simulink model "poly3DoublyNormalized"  (R2023b)
settings: Solver=FixedStepAuto  StartTime=0.0  StopTime=10  FixedStep=0.0001  MaxStep=0.001  RelTol=1e-3
settings Model: Creator=ggi01  LastModifiedBy=ggi01
settings SolverCC: AlgebraicLoopSolver=TrustRegion
settings DebuggingCC: UnconnectedInputMsg=warning  UnconnectedOutputMsg=warning  UnconnectedLineMsg=warning
settings ModelReferenceCC: EnableRefExpFcnMdlSchedulingChecks=on
settings RTWCC: DLArmComputeVersion=19.05

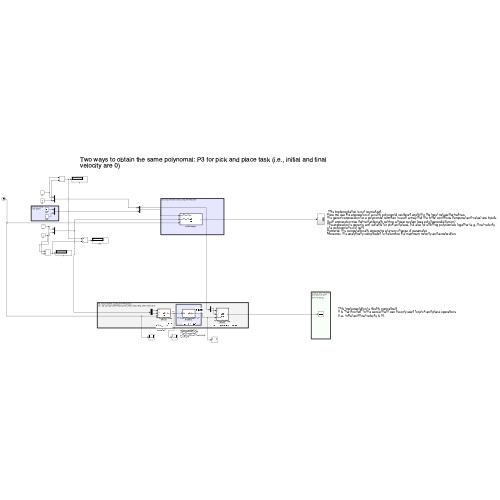
[thumbnail: Simulink's stored preview of the top-level diagram]
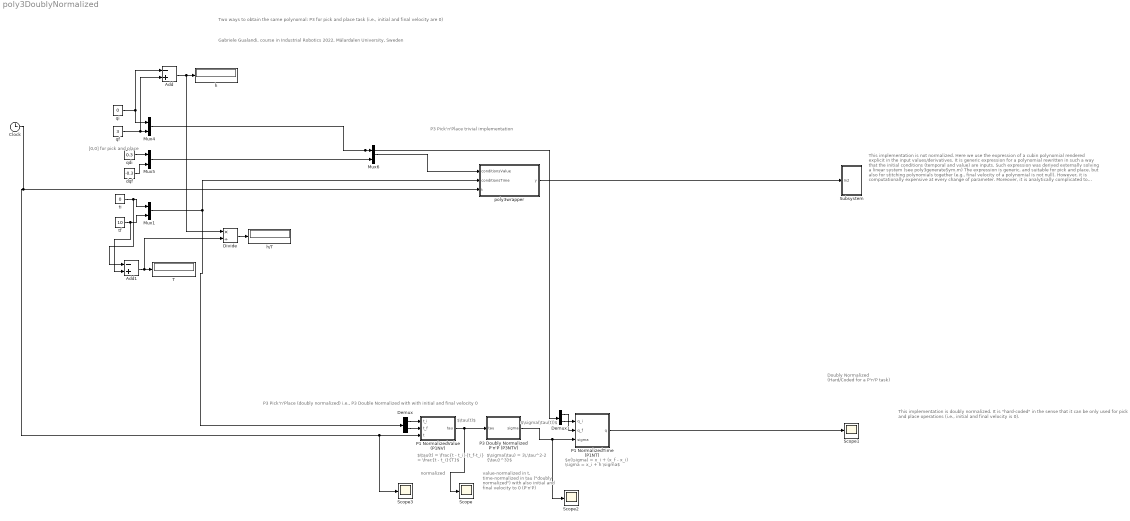
== system poly3DoublyNormalized ==
  note: P3 Pick'n'Place trivial implementation
  note: Gabriele Gualandi, course in Industrial Robotics 2022, Mälardalen University, Sweden
  note: normalized
  note: Two ways to obtain the same polynomal: P3 for pick and place task (i.e., initial and final velocity are 0)
  note: [0,0] for pick
      | and place
  note: P3 Pick'n'Place (doubly normalized)
      | i.e., P3 Double Normalized with with initial and final velocity 0
  note: Doubly Normalized
      | (Hard/Coded for
      | a P'n'P task)
  note: This implementation is not normalized.
      | Here we use the expression of a cubin polynomial rendered explicit in the input values/derivatives.
      | It is generic expression for a polynomial rewritten in such a way that the initial conditions (temporal and value) are inputs. Such expression was derived externally solving a linear system (see poly3generateSym.m)
      | The expression is generic, and suitable for pick and place, but also for stitching polynomials together (e.g., final velocity of a polynomial is not null).
      | However, it is computationally expensive at every change of parameter.
      | Moreover, it is analytically complicated to determine the maximum velocity and acceleration.
  note: This implementation is doubly normalized.
      | It is "hard-coded" in the sense that it can be only used for pick and place operations
      | (i.e., initial and final velocity is 0).
  note: $\sigma(\tau) = 3\,\tau^2-2 {\tau}^3}$
  note: $\tau(t)$
  note: value-normalized in t,
      | time-normalized in tau
      | ("doubly normalized")
      | with also initial and final velocity
      | to 0 (P'n'P)
  note: $\sigma(\tau(t))$
  note: $\tau(t) = \frac{t - t_i}{t_f-t_i} = \frac{t - t_i}{T}$
  note: $x(\sigma) = x_i + (x_f - x_i) \sigma = x_i + h \sigma$
  Add : Sum  Inputs=-+
  Add1 : Sum  Inputs=-+
  Clock : Clock
  Demux : Demux  Outputs=2
  Demux1 : Demux  Outputs=2
  Divide : Product  Inputs=*/
  Mux{1,4..6} (4 alike) : Mux  Inputs=2
  P1 NormalizedTime (P1NT) : MATLAB Function  TreatAsAtomicUnit=on
  P1 NormalizedValue (P1NV) : MATLAB Function  TreatAsAtomicUnit=on
  P3 Doubly Normalized P'n'P (P3NTV) : MATLAB Function  TreatAsAtomicUnit=on
  Scope{,1..3} (4 alike) : Scope
  Subsystem : Subsystem
  T : Display
  dqf : Constant  Value=-0.3
  h : Display
  h/T : Display
  poly3wrapper : MATLAB Function  TreatAsAtomicUnit=on
  qdi : Constant  Value=0.3
  qf : Constant  Value=3
  qi : Constant  Value=0
  tf : Constant  Value=10
  ti : Constant  Value=0
  wires:
  qi/1 -> Mux4/1, Add/1
  qf/1 -> Add/2, Mux4/2
  qdi/1 -> Mux5/1
  dqf/1 -> Mux5/2
  ti/1 -> Add1/1, Mux1/1
  tf/1 -> Add1/2, Mux1/2
  Mux1/1 -> Demux/1, poly3wrapper/2(conditionsTime)
  Mux4/1 -> Demux1/1, Mux6/1
  Mux6/1 -> poly3wrapper/1(conditionsValue)
  Mux5/1 -> Mux6/2
  Demux/1 -> P1 NormalizedValue (P1NV)/1(t_i)
  Demux/2 -> P1 NormalizedValue (P1NV)/2(t_f)
  Demux1/1 -> P1 NormalizedTime (P1NT)/1(q_i)
  Demux1/2 -> P1 NormalizedTime (P1NT)/2(q_f)
  P1 NormalizedTime (P1NT)/1(q) -> Scope1/1
  P1 NormalizedValue (P1NV)/1(tau) -> Scope/1, P3 Doubly Normalized P'n'P (P3NTV)/1(tau)
  P3 Doubly Normalized P'n'P (P3NTV)/1(sigma) -> Scope2/1, P1 NormalizedTime (P1NT)/3(sigma)
  Clock/1 -> Scope3/1, P1 NormalizedValue (P1NV)/3(t), poly3wrapper/3(t)
  poly3wrapper/1(y) -> Subsystem/1(In2)
  Add/1 -> Divide/1, h/1
  Add1/1 -> Divide/2, T/1
  Divide/1 -> h/T/1

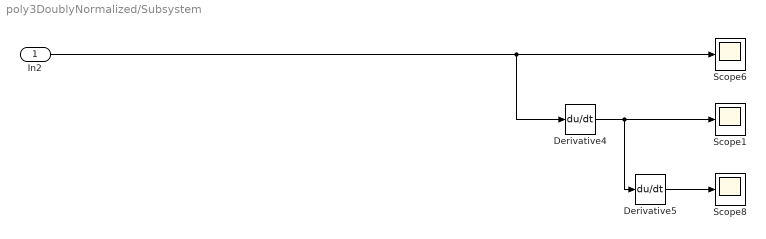
== system poly3DoublyNormalized/Subsystem ==
  In2 : Inport
  Derivative4 : Derivative
  Derivative5 : Derivative
  Scope1 : Scope
  Scope6 : Scope
  Scope8 : Scope
  wires:
  Derivative5/1 -> Scope8/1
  In2/1 -> Scope6/1, Derivative4/1
  Derivative4/1 -> Scope1/1, Derivative5/1

== matlab function poly3DoublyNormalized/P3 Doubly Normalized P'n'P (P3NTV) ==
  data: tau input; sigma output
function sigma = fcn(tau)

sigma = 3 * tau^2 - 2 * tau^3;

== matlab function poly3DoublyNormalized/P1 NormalizedTime (P1NT) ==
  data: q_i input; q output; q_f input; sigma input
function q = fcn(q_i,q_f,sigma)

h = q_f - q_i;
q = q_i + h * sigma;

== matlab function poly3DoublyNormalized/poly3wrapper ==
  data: conditionsValue input; y output; conditionsTime input; t input
function y = fcn(conditionsValue, conditionsTime, t)
    y = poly3(conditionsValue,conditionsTime,t);

== matlab function poly3DoublyNormalized/P1 NormalizedValue (P1NV) ==
  data: t_i input; t_f input; t input; tau output
function tau = t2tau(t_i,t_f,t)
T = t_f - t_i;
tau = (t - t_i)/T;
